simulink model "chap3_eoct_1_3"  (R2018b)
settings: Solver=VariableStepAuto  StartTime=0.0  StopTime=Endtime  RelTol=1e-3
values from neighbouring files (symbols this model uses):
  a = 5    [chap3_1_3.m]
  C = D ^2 / 4 *pi    (= 0.196349540849)    [chap3_1_3.m]
  q1_delta = 1*10^(-5)    (= 1e-05)    [chap3_1_3.m]
  R = 500    [chap3_1_3.m]
libraries: simulink x1
settings Model: Creator=nharada  LastModifiedBy=nharada

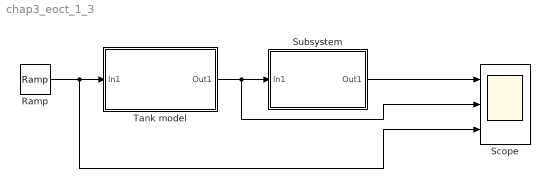
== system chap3_eoct_1_3 ==
  Ramp : simulink/Sources/Ramp  slope=q1_delta  start=st  InitialOutput=0
  Scope : Scope  NumInputPorts=3
  Subsystem : Subsystem
  "Tank model " : Subsystem
  wires:
  Ramp/1 -> "Tank model "/1(In1), Scope/3
  Subsystem/1(Out1) -> Scope/1
  "Tank model "/1(Out1) -> Scope/2, Subsystem/1(In1)

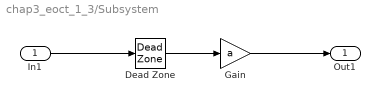
== system chap3_eoct_1_3/Subsystem ==
  In1 : Inport
  Dead Zone : DeadZone  LowerValue=-inf  UpperValue=d  SaturateOnIntegerOverflow=on
  Gain : Gain  Gain=a
  Out1 : Outport
  wires:
  Dead Zone/1 -> Gain/1
  In1/1 -> Dead Zone/1
  Gain/1 -> Out1/1

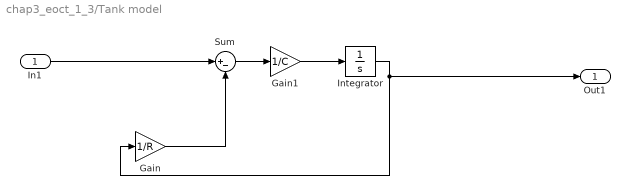
== system chap3_eoct_1_3/Tank model  ==
  In1 : Inport
  Gain : Gain  Gain=1/R
  Gain1 : Gain  Gain=1/C
  Integrator : Integrator
  Sum : Sum  Inputs=|+-
  Out1 : Outport
  wires:
  In1/1 -> Sum/1
  Gain1/1 -> Integrator/1
  Integrator/1 -> Out1/1, Gain/1
  Sum/1 -> Gain1/1
  Gain/1 -> Sum/2
